simulink model "observador"  (R2020b)
settings: Solver=VariableStepAuto  StartTime=0.0  StopTime=40  RelTol=1e-3
settings Model: Creator=petir  LastModifiedBy=petir

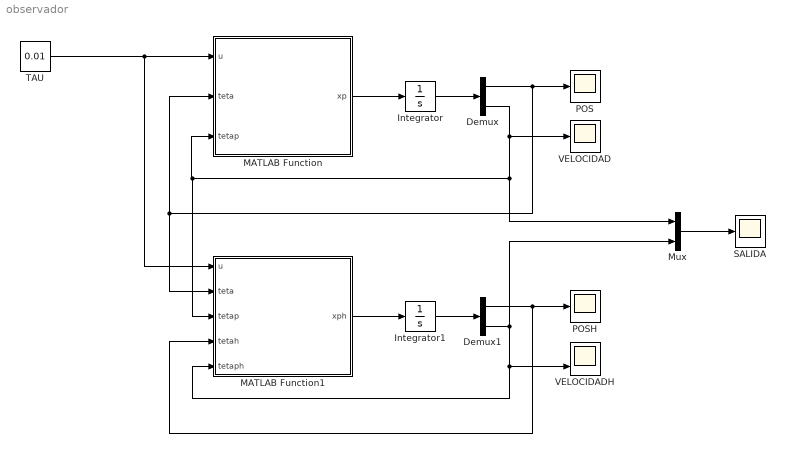
== system observador ==
  Demux : Demux  Outputs=2
  Demux1 : Demux  Outputs=2
  Integrator : Integrator
  Integrator1 : Integrator
  MATLAB Function : MATLAB Function  TreatAsAtomicUnit=on
  MATLAB Function1 : MATLAB Function  TreatAsAtomicUnit=on
  Mux : Mux  Inputs=2
  POS : Scope
  POSH : Scope
  SALIDA : Scope
  TAU : Constant  Value=0.01
  VELOCIDAD : Scope
  VELOCIDADH : Scope  NumInputPorts=2
  wires:
  Integrator/1 -> Demux/1
  MATLAB Function/1(xp) -> Integrator/1
  Demux/2 -> VELOCIDAD/1, Mux/1, MATLAB Function1/3(tetap), MATLAB Function/3(tetap)
  Demux/1 -> POS/1, MATLAB Function/2(teta), MATLAB Function1/2(teta)
  Demux1/2 -> Mux/2, MATLAB Function1/5(tetaph), VELOCIDADH/2
  MATLAB Function1/1(xph) -> Integrator1/1
  Demux1/1 -> MATLAB Function1/4(tetah), POSH/1
  Integrator1/1 -> Demux1/1
  TAU/1 -> MATLAB Function1/1(u), MATLAB Function/1(u)
  Mux/1 -> SALIDA/1

== matlab function observador/MATLAB Function1 ==
  data: u input; xph output; teta input; tetap input; tetah input; tetaph input
function xph = fcn(u, teta, tetap, tetah, tetaph)
% Parámetros
J = 80.7e-6;
B1 = 14.41e-6;
K = [19.8214; 96.8214]

A = [0, 1; 0, -B1/J];
B = [0; 1/J];
C = [1, 0];

% Observador
xh = [tetah; tetaph];
x = [teta; tetap];
y = C * x;
yh = C *xh;
xph = A * xh + B * u + K *(y - yh);

== matlab function observador/MATLAB Function ==
  data: u input; xp output; teta input; tetap input
function xp = fcn(u, teta, tetap)
% Parámetros
J = 80.7e-6;
B1 = 14.41e-6;

A = [0, 1; 0, -B1/J];
B = [0; 1/J];
% C = [1, 0];

% Planta
x = [teta; tetap]
xp = A * x + B*u;
